simulink model "PM"  (R2020b)
settings: Solver=VariableStepAuto  StartTime=0.0  StopTime=10.0  RelTol=1e-3
settings Model: Creator=MEDIA  LastModifiedBy=MEDIA

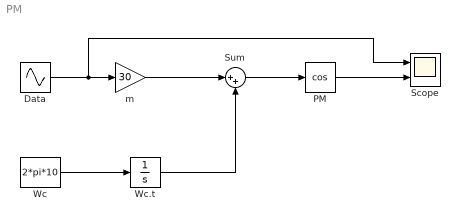
== system PM ==
  Data : Sin  Frequency=2*pi  SampleTime=1/5000
  PM : Trigonometry  Operator=cos
  Scope : Scope  NumInputPorts=2
  Sum : Sum  Inputs=|++
  Wc : Constant  Value=2*pi*10
  Wc.t : Integrator
  m : Gain  Gain=30
  wires:
  Data/1 -> Scope/1, m/1
  m/1 -> Sum/1
  Wc/1 -> Wc.t/1
  Wc.t/1 -> Sum/2
  Sum/1 -> PM/1
  PM/1 -> Scope/2
